simulink model "stellaris_test_uart_nb"  (R2012b)
settings: Solver=FixedStepDiscrete  SolverMode=SingleTasking  StartTime=0.0  StopTime=10.0  FixedStep=0.2  RelTol=1e-3
libraries: stellaris_lib x2, simulink x1
settings Model: Creator=peselnikmg  LastModifiedBy=peselnikmg
settings DataIOCC: SignalLoggingSaveFormat=ModelDataLogs
settings OptimizationCC: OptimizeModelRefInitCode=on  LifeSpan=1
settings HardwareCC: ProdEndianess=LittleEndian  ProdHWDeviceType=Texas Instruments->TMS470
settings RTWCC: SystemTargetFile=stellaris.tlc  TemplateMakefile=stellaris_tmf  PostCodeGenCommand=stellaris_customcode(buildInfo)  Description=TI Stellaris LaunchPad  GenerateReport=on  ProcessScript=stellaris_make_rtw_hook  IncludeHyperlinkInReport=on  GenerateTraceInfo=on  GenerateTraceReport=on  GenerateTraceReportSl=on  GenerateTraceReportSf=on  GenerateTraceReportEml=on  GenerateCodeMetricsReport=on  GenerateCodeReplacementReport=on
settings CodeAppCC: IgnoreCustomStorageClasses=off
settings STFCustomTargetCC: CodeReplacementLibrary=ANSI_C  CombineOutputUpdateFcns=on  ERTCustomFileBanners=on  SupportContinuousTime=off  SupportNonInlinedSFcns=off  GRTInterface=off  SystemTargetFile=stellaris.tlc
settings ERTTargetCC: CodeReplacementLibrary=ANSI_C  MultiwordLength=2048  ParMdlRefBuildCompliant=off  CompOptLevelCompliant=off  ConcurrentExecutionCompliant=off  ERTFirstTimeCompliant=off  ModelStepFunctionPrototypeControlCompliant=off  CPPClassGenCompliant=off  InlinedParameterPlacement=NonHierarchical  ERTCustomFileTemplate=stellaris_srmain.tlc  ConvertIfToSwitch=off  SuppressUnreachableDefaultCases=off

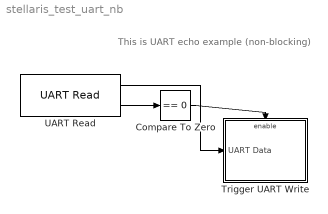
== system stellaris_test_uart_nb ==
  note: This is UART echo example (non-blocking)
  Compare To Zero : simulink/Logic and Bit Operations/Compare To Zero  relop===  OutDataTypeStr=boolean
  Trigger UART Write : Subsystem
  UART Read : stellaris_lib/UART/UART Read  nbFlag=on
  wires:
  UART Read/1 -> Trigger UART Write/1(UART Data)
  UART Read/2 -> Compare To Zero/1
  Compare To Zero/1 -> Trigger UART Write/Enable

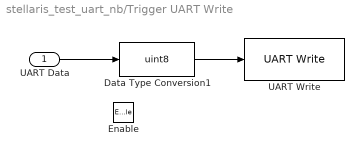
== system stellaris_test_uart_nb/Trigger UART Write ==
  UART Data : Inport
  Enable : EnablePort
  Data Type Conversion1 : DataTypeConversion  OutDataTypeStr=uint8
  UART Write : stellaris_lib/UART/UART Write  nbFlag=on
  wires:
  Data Type Conversion1/1 -> UART Write/1
  UART Data/1 -> Data Type Conversion1/1
